simulink model "TEP_Final_NoScript"  (R2024a)
settings: Solver=FixedStepAuto  StartTime=0.0  StopTime=10  FixedStep=1/3600  RelTol=1e-3
model workspace (MAT data in the model file):
  AD : Simulink.Parameter (value not decoded)
  AG : Simulink.Parameter (value not decoded)
  AH : Simulink.Parameter (value not decoded)
  AV : Simulink.Parameter (value not decoded)
  AVP : Simulink.Parameter (value not decoded)
  BCHL : Simulink.Parameter (value not decoded)
  BCHV : Simulink.Parameter (value not decoded)
  BD : Simulink.Parameter (value not decoded)
  BG : Simulink.Parameter (value not decoded)
  BH : Simulink.Parameter (value not decoded)
  BVP : Simulink.Parameter (value not decoded)
  CD : Simulink.Parameter (value not decoded)
  CG : Simulink.Parameter (value not decoded)
  CH : Simulink.Parameter (value not decoded)
  CVP : Simulink.Parameter (value not decoded)
  XMW : Simulink.Parameter (value not decoded)
  XNS : Simulink.Parameter (value not decoded)
  XNSE : Simulink.Parameter (value not decoded)
symbols that are objects in the model workspace (value not decoded): AD, AG, AH, AV, AVP, BD, BG, BH, BVP, CD, CG, CH, CVP, XMW, XNS, XNSE
undefined symbols (not defined in the file or in its folder): magnitude, msgbox, SETPT, XMEAS, XMV
libraries: mylib x360, dspindex x28
(part 8 of 14)

== system TEP_Final_NoScript/Subsystem1/CCin/Subsystem3 ==
  TC : Inport
  P : Inport  Port=2
  Add : Sum  Inputs=+-
  P0 Pa : Constant  Value=1.01325e5
  Subsystem : Subsystem
  Subsystem1 : Subsystem
  Subsystem2 : Subsystem
  T0 K : Constant  Value=298.15
  kPa to Pa : Gain  Gain=1000
  Bph : Outport
  wires:
  kPa to Pa/1 -> Subsystem1/3(P1)
  P0 Pa/1 -> Subsystem1/4(P0)
  Subsystem/1(h-h0 J/mol) -> Add/1
  Subsystem1/1(T0(s-s0) J/mol) -> Add/2
  T0 K/1 -> Subsystem1/2(T0), Subsystem/2(T0)
  Subsystem2/1(TK) -> Subsystem/1(T1), Subsystem1/1(T1)
  TC/1 -> Subsystem2/1(TC)
  Add/1 -> Bph/1
  P/1 -> kPa to Pa/1

== system TEP_Final_NoScript/Subsystem1/CCout/Subsystem ==
  Bph : Inport
  FWR in kg/h : Inport  Port=2
  Gain : Gain  Gain=1/3600
  Product : Product
  kg/kmol : Constant  Value=18.02
  kmol to mol : Gain  Gain=1000
  kmol/h : Product  Inputs=*/
  Bphm J/s : Outport  VectorParamsAs1DForOutWhenUnconnected=off
  wires:
  Product/1 -> Gain/1
  kmol/h/1 -> kmol to mol/1
  Bph/1 -> Product/1
  Gain/1 -> Bphm J/s/1
  kg/kmol/1 -> kmol/h/2
  FWR in kg/h/1 -> kmol/h/1
  kmol to mol/1 -> Product/2

== system TEP_Final_NoScript/Subsystem1/CCout/Subsystem1 ==
  T : Inport
  F : Inport  Port=2
  A : Constant  Value=9.069
  Gain : Gain  Gain=1/3600
  J/mol : Product
  Product : Product
  Product1 : Product
  gpm to lb/h : Constant  Value=500.72
  lb/h to lb-mol/h : Product  Inputs=*/
  lb/lb-mol : Constant  Value=18.02
  mol : Constant  Value=453.59
  mol/h : Product
  Q J/s : Outport  VectorParamsAs1DForOutWhenUnconnected=off
  wires:
  A/1 -> J/mol/1
  mol/1 -> mol/h/1
  lb/lb-mol/1 -> lb/h to lb-mol/h/2
  Product1/1 -> lb/h to lb-mol/h/1
  lb/h to lb-mol/h/1 -> mol/h/2
  Product/1 -> Gain/1
  gpm to lb/h/1 -> Product1/2
  Gain/1 -> Q J/s/1
  mol/h/1 -> Product/2
  J/mol/1 -> Product/1
  T/1 -> J/mol/2
  F/1 -> Product1/1

== system TEP_Final_NoScript/Subsystem1/CCout/Subsystem3 ==
  TC : Inport
  P : Inport  Port=2
  Add : Sum  Inputs=+-
  P0 Pa : Constant  Value=1.01325e5
  Subsystem : Subsystem
  Subsystem1 : Subsystem
  Subsystem2 : Subsystem
  T0 K : Constant  Value=298.15
  kPa to Pa : Gain  Gain=1000
  Bph : Outport
  wires:
  kPa to Pa/1 -> Subsystem1/3(P1)
  P0 Pa/1 -> Subsystem1/4(P0)
  Subsystem/1(h-h0 J/mol) -> Add/1
  Subsystem1/1(T0(s-s0) J/mol) -> Add/2
  T0 K/1 -> Subsystem1/2(T0), Subsystem/2(T0)
  Subsystem2/1(TK) -> Subsystem/1(T1), Subsystem1/1(T1)
  TC/1 -> Subsystem2/1(TC)
  Add/1 -> Bph/1
  P/1 -> kPa to Pa/1

== system TEP_Final_NoScript/Subsystem1/D feed stream/Composition measurement mol% ==
  XST : Inport
  XMNSE : Inport  Port=2
  Bus Creator : BusCreator  Inputs=8
  Subsystem : Subsystem
  SMEASX : Outport
  wires:
  Subsystem/4(SMEASXD) -> Bus Creator/4  "SMEASXD"
  Subsystem/5(SMEASXE) -> Bus Creator/5  "SMEASXE"
  Subsystem/6(SMEASXF) -> Bus Creator/6  "SMEASXF"
  Subsystem/7(SMEASXG) -> Bus Creator/7  "SMEASXG"
  Subsystem/8(SMEASXH) -> Bus Creator/8  "SMEASXH"
  Subsystem/3(SMEASXC) -> Bus Creator/3  "SMEASXC"
  XST/1 -> Subsystem/1(XST)
  Subsystem/2(SMEASXB) -> Bus Creator/2  "SMEASXB"
  Subsystem/1(SMEASXA) -> Bus Creator/1  "SMEASXA"
  Bus Creator/1 -> SMEASX/1  "SMEASX"
  XMNSE/1 -> Subsystem/2(XMNSE)

== system TEP_Final_NoScript/Subsystem1/D feed stream/Flow measurement in kg//h ==
  XMEAS in kg/h : Inport
  "SMEASF " : Outport  VectorParamsAs1DForOutWhenUnconnected=off
  wires:
  XMEAS in kg/h/1 -> "SMEASF "/1

== system TEP_Final_NoScript/Subsystem1/D feed stream/Pressure measurement in kPa ==
  "P in mm Hg " : Inport
  XMNSE : Inport  Port=2
  " kPa" : Constant  Value=101.325
  " mm Hg   " : Constant  Value=760
  Add : Sum
  Pressure conversion kPa : Product  Inputs=*/*
  SMEASP : Outport  VectorParamsAs1DForOutWhenUnconnected=off
  wires:
  "P in mm Hg "/1 -> Pressure conversion kPa/1
  " kPa"/1 -> Pressure conversion kPa/3
  " mm Hg   "/1 -> Pressure conversion kPa/2
  Pressure conversion kPa/1 -> Add/1
  Add/1 -> SMEASP/1  "SMEASP"
  XMNSE/1 -> Add/2

== system TEP_Final_NoScript/Subsystem1/D feed stream/Temperature measurement in C ==
  T in celsius : Inport
  XMNSE : Inport  Port=2
  Add : Sum
  SMEAST : Outport
  wires:
  T in celsius/1 -> Add/1
  Add/1 -> SMEAST/1  "SMEAST"
  XMNSE/1 -> Add/2

== system TEP_Final_NoScript/Subsystem1/E feed stream/Composition measurement mol% ==
  XST : Inport
  XMNSE : Inport  Port=2
  Bus Creator : BusCreator  Inputs=8
  Subsystem : Subsystem
  SMEASX : Outport
  wires:
  Subsystem/4(SMEASXD) -> Bus Creator/4  "SMEASXD"
  Subsystem/5(SMEASXE) -> Bus Creator/5  "SMEASXE"
  Subsystem/6(SMEASXF) -> Bus Creator/6  "SMEASXF"
  Subsystem/7(SMEASXG) -> Bus Creator/7  "SMEASXG"
  Subsystem/8(SMEASXH) -> Bus Creator/8  "SMEASXH"
  Subsystem/3(SMEASXC) -> Bus Creator/3  "SMEASXC"
  XST/1 -> Subsystem/1(XST)
  Subsystem/2(SMEASXB) -> Bus Creator/2  "SMEASXB"
  Subsystem/1(SMEASXA) -> Bus Creator/1  "SMEASXA"
  Bus Creator/1 -> SMEASX/1  "SMEASX"
  XMNSE/1 -> Subsystem/2(XMNSE)

== system TEP_Final_NoScript/Subsystem1/E feed stream/Flow measurement in kg//h ==
  XMEAS in kg/h : Inport
  "SMEASF " : Outport  VectorParamsAs1DForOutWhenUnconnected=off
  wires:
  XMEAS in kg/h/1 -> "SMEASF "/1

== system TEP_Final_NoScript/Subsystem1/E feed stream/Pressure measurement in kPa ==
  "P in mm Hg " : Inport
  XMNSE : Inport  Port=2
  " kPa" : Constant  Value=101.325
  " mm Hg   " : Constant  Value=760
  Add : Sum
  Pressure conversion kPa : Product  Inputs=*/*
  SMEASP : Outport  VectorParamsAs1DForOutWhenUnconnected=off
  wires:
  "P in mm Hg "/1 -> Pressure conversion kPa/1
  " kPa"/1 -> Pressure conversion kPa/3
  " mm Hg   "/1 -> Pressure conversion kPa/2
  Pressure conversion kPa/1 -> Add/1
  Add/1 -> SMEASP/1  "SMEASP"
  XMNSE/1 -> Add/2

== system TEP_Final_NoScript/Subsystem1/E feed stream/Temperature measurement in C ==
  T in celsius : Inport
  XMNSE : Inport  Port=2
  Add : Sum
  SMEAST : Outport
  wires:
  T in celsius/1 -> Add/1
  Add/1 -> SMEAST/1  "SMEAST"
  XMNSE/1 -> Add/2

== system TEP_Final_NoScript/Subsystem1/Product stream/Composition measurement mol% ==
  XST : Inport
  XMNSE2 : Inport  Port=2
  XMNSE3 : Inport  Port=3
  Bus Creator : BusCreator  Inputs=8
  Subsystem : Subsystem
  Subsystem1 : Subsystem
  SMEASX : Outport
  wires:
  Subsystem/3(SMEASXC) -> Bus Creator/3  "SMEASXC"
  XST/1 -> Subsystem1/1(XST), Subsystem/1(XST)
  Subsystem/2(SMEASXB) -> Bus Creator/2  "SMEASXB"
  Subsystem/1(SMEASXA) -> Bus Creator/1  "SMEASXA"
  Bus Creator/1 -> SMEASX/1  "SMEASX"
  XMNSE2/1 -> Subsystem/2(XMNSE)
  Subsystem1/1(SMEASXD) -> Bus Creator/4  "SMEASXD"
  Subsystem1/2(SMEASXE) -> Bus Creator/5  "SMEASXE"
  Subsystem1/3(SMEASXF) -> Bus Creator/6  "SMEASXF"
  Subsystem1/4(SMEASXG) -> Bus Creator/7  "SMEASXG"
  Subsystem1/5(SMEASXH) -> Bus Creator/8  "SMEASXH"
  XMNSE3/1 -> Subsystem1/2(XMNSE3)

== system TEP_Final_NoScript/Subsystem1/Product stream/Flow measurement in kg//h ==
  XMEAS in m^3/h : Inport
  XST : Inport  Port=2
  "       " : Constant  Value=35.3145
  Convert from lb/h to kg/h : Constant  Value=0.454
  XMWS Molecular weight of Stream lb/lb-mol : Subsystem
  kg/h : Product  Inputs=3
  lb-mol/h : Product  Inputs=***
  "SMEASF " : Outport  VectorParamsAs1DForOutWhenUnconnected=off
  wires:
  lb-mol/h/1 -> kg/h/2
  [DLS] -> lb-mol/h/2
  "       "/1 -> lb-mol/h/3
  XMEAS in m^3/h/1 -> lb-mol/h/1
  XMWS Molecular weight of Stream lb/lb-mol/1(XMWS) -> kg/h/1
  Convert from lb/h to kg/h/1 -> kg/h/3
  kg/h/1 -> "SMEASF "/1
  XST/1 -> XMWS Molecular weight of Stream lb/lb-mol/1(XST)

== system TEP_Final_NoScript/Subsystem1/Product stream/Pressure measurement in kPa ==
  "P in mm Hg " : Inport
  XMNSE : Inport  Port=2
  " kPa" : Constant  Value=101.325
  " mm Hg   " : Constant  Value=760
  Add : Sum
  Pressure conversion kPa : Product  Inputs=*/*
  SMEASP : Outport  VectorParamsAs1DForOutWhenUnconnected=off
  wires:
  "P in mm Hg "/1 -> Pressure conversion kPa/1
  " kPa"/1 -> Pressure conversion kPa/3
  " mm Hg   "/1 -> Pressure conversion kPa/2
  Pressure conversion kPa/1 -> Add/1
  Add/1 -> SMEASP/1  "SMEASP"
  XMNSE/1 -> Add/2

== system TEP_Final_NoScript/Subsystem1/Product stream/Temperature measurement in C ==
  XMEAS in celsius : Inport
  SMEAST : Outport
  wires:
  XMEAS in celsius/1 -> SMEAST/1  "SMEAST"

== system TEP_Final_NoScript/Subsystem1/Purge stream/Composition measurement mol% ==
  XMEAS : Inport
  Bus Creator : BusCreator  Inputs=8
  Bus Selector : BusSelector  OutputSignals=XMEAS(29),XMEAS(30),XMEAS(31),XMEAS(32),XMEAS(33),XMEAS(34),XMEAS(35),XMEAS(36)
  SMEASX : Outport
  wires:
  Bus Selector/4 -> Bus Creator/4  "<XMEAS(32)>"
  Bus Selector/5 -> Bus Creator/5  "<XMEAS(33)>"
  Bus Selector/6 -> Bus Creator/6  "<XMEAS(34)>"
  Bus Selector/7 -> Bus Creator/7  "<XMEAS(35)>"
  Bus Selector/8 -> Bus Creator/8  "<XMEAS(36)>"
  Bus Selector/3 -> Bus Creator/3  "<XMEAS(31)>"
  XMEAS/1 -> Bus Selector/1
  Bus Selector/2 -> Bus Creator/2  "<XMEAS(30)>"
  Bus Selector/1 -> Bus Creator/1  "<XMEAS(29)>"
  Bus Creator/1 -> SMEASX/1  "SMEASX"

== system TEP_Final_NoScript/Subsystem1/Purge stream/Flow measurement in kg//h ==
  XMEAS in kscmh : Inport
  XST : Inport  Port=2
  " " : Constant  Value=35.3145
  "  " : Constant  Value=0.359
  Convert from lb/h to kg/h : Constant  Value=0.454
  Product : Product  Inputs=3
  XMWS Molecular weight of Stream lb/lb-mol : Subsystem
  lb-mol/h : Product  Inputs=**/
  "SMEASF " : Outport  VectorParamsAs1DForOutWhenUnconnected=off
  wires:
  " "/1 -> lb-mol/h/2
  "  "/1 -> lb-mol/h/3
  XMEAS in kscmh/1 -> lb-mol/h/1
  Convert from lb/h to kg/h/1 -> Product/3
  XST/1 -> XMWS Molecular weight of Stream lb/lb-mol/1(XST)
  lb-mol/h/1 -> Product/2
  XMWS Molecular weight of Stream lb/lb-mol/1(XMWS) -> Product/1
  Product/1 -> "SMEASF "/1

== system TEP_Final_NoScript/Subsystem1/Purge stream/Pressure measurement in kPa ==
  XMEAS in kPa gauge : Inport
  " kPa" : Constant  Value=101.325
  Add : Sum
  SMEASP : Outport  VectorParamsAs1DForOutWhenUnconnected=off
  wires:
  Add/1 -> SMEASP/1  "SMEASP"
  " kPa"/1 -> Add/2
  XMEAS in kPa gauge/1 -> Add/1

== system TEP_Final_NoScript/Subsystem1/Purge stream/Temperature measurement in C ==
  XMEAS in celsius : Inport
  SMEAST : Outport
  wires:
  XMEAS in celsius/1 -> SMEAST/1  "SMEAST"

== system TEP_Final_NoScript/Subsystem1/RCIn/Flow measurement in kg//h ==
  XMNSE : Inport
  F in gpm : Inport  Port=2
  Add : Sum
  Product : Product
  Product1 : Product
  gpm to lb/h : Constant  Value=500.72
  kg/kmol : Constant  Value=18.02
  kmol : Constant  Value=0.45359237
  kmol/h : Product
  lb/h to lb-mol/h : Product  Inputs=*/
  lb/lb-mol : Constant  Value=18.02
  "SMEASF " : Outport  VectorParamsAs1DForOutWhenUnconnected=off
  wires:
  Add/1 -> "SMEASF "/1  "SMEASF"
  Product/1 -> Add/1
  XMNSE/1 -> Add/2
  Product1/1 -> lb/h to lb-mol/h/1
  lb/lb-mol/1 -> lb/h to lb-mol/h/2
  lb/h to lb-mol/h/1 -> kmol/h/2
  gpm to lb/h/1 -> Product1/2
  F in gpm/1 -> Product1/1
  kmol/1 -> kmol/h/1
  kmol/h/1 -> Product/1
  kg/kmol/1 -> Product/2

== system TEP_Final_NoScript/Subsystem1/RCIn/Pressure measurement in kPa ==
  XMNSE : Inport
  TC : Inport  Port=2
  A Antoine Coefficient A : Constant  Value=11.6834
  Add : Sum
  Add1 : Sum
  Add2 : Sum  Inputs=+-
  B Antoine Coefficient B : Constant  Value=3816.44
  C Antoine Coefficient C : Constant  Value=-46.13
  Divide : Product  Inputs=*/
  Divide1 : Product  Inputs=**
  Math Function : Math  SignedPower=on
  Temperature in Kelvin K : Sum
  To Convert bar to kPa : Constant  Value=100
  To Convert °C to K : Constant  Value=273.15
  SMEASP : Outport  VectorParamsAs1DForOutWhenUnconnected=off
  wires:
  Add/1 -> SMEASP/1  "SMEASP"
  XMNSE/1 -> Add/2
  To Convert °C to K/1 -> Temperature in Kelvin K/2
  TC/1 -> Temperature in Kelvin K/1
  C Antoine Coefficient C/1 -> Add1/1
  Divide/1 -> Add2/2
  B Antoine Coefficient B/1 -> Divide/1
  Add1/1 -> Divide/2
  Math Function/1 -> Divide1/1
  A Antoine Coefficient A/1 -> Add2/1
  Add2/1 -> Math Function/1
  To Convert bar to kPa/1 -> Divide1/2
  Temperature in Kelvin K/1 -> Add1/2
  Divide1/1 -> Add/1

== system TEP_Final_NoScript/Subsystem1/RCIn/Temperature measurement in C ==
  T in celsius : Inport
  XMNSE : Inport  Port=2
  Add : Sum
  SMEAST : Outport
  wires:
  T in celsius/1 -> Add/1
  Add/1 -> SMEAST/1  "SMEAST"
  XMNSE/1 -> Add/2

== system TEP_Final_NoScript/Subsystem1/RCOut/Pressure measurement in kPa ==
  XMNSE : Inport
  TC : Inport  Port=2
  A Antoine Coefficient A : Constant  Value=11.6834
  Add : Sum
  Add1 : Sum
  Add2 : Sum  Inputs=+-
  B Antoine Coefficient B : Constant  Value=3816.44
  C Antoine Coefficient C : Constant  Value=-46.13
  Divide : Product  Inputs=*/
  Divide1 : Product  Inputs=**
  Math Function : Math  SignedPower=on
  Temperature in Kelvin K : Sum
  To Convert bar to kPa : Constant  Value=100
  To Convert °C to K : Constant  Value=273.15
  SMEASP : Outport  VectorParamsAs1DForOutWhenUnconnected=off
  wires:
  Add/1 -> SMEASP/1  "SMEASP"
  XMNSE/1 -> Add/2
  To Convert °C to K/1 -> Temperature in Kelvin K/2
  TC/1 -> Temperature in Kelvin K/1
  C Antoine Coefficient C/1 -> Add1/1
  Divide/1 -> Add2/2
  B Antoine Coefficient B/1 -> Divide/1
  Add1/1 -> Divide/2
  Math Function/1 -> Divide1/1
  A Antoine Coefficient A/1 -> Add2/1
  Add2/1 -> Math Function/1
  To Convert bar to kPa/1 -> Divide1/2
  Temperature in Kelvin K/1 -> Add1/2
  Divide1/1 -> Add/1

== system TEP_Final_NoScript/Subsystem1/RCOut/Temperature measurement in C ==
  T in celsius : Inport
  XMNSE : Inport  Port=2
  Add : Sum
  SMEAST : Outport
  wires:
  T in celsius/1 -> Add/1
  Add/1 -> SMEAST/1  "SMEAST"
  XMNSE/1 -> Add/2

== system TEP_Final_NoScript/Subsystem1/RCin/Subsystem ==
  Bph : Inport
  FWR in kg/h : Inport  Port=2
  Gain : Gain  Gain=1/3600
  Product : Product
  kg/kmol : Constant  Value=18.02
  kmol to mol : Gain  Gain=1000
  kmol/h : Product  Inputs=*/
  Bphm J/s : Outport  VectorParamsAs1DForOutWhenUnconnected=off
  wires:
  Product/1 -> Gain/1
  kmol/h/1 -> kmol to mol/1
  Bph/1 -> Product/1
  Gain/1 -> Bphm J/s/1
  kg/kmol/1 -> kmol/h/2
  FWR in kg/h/1 -> kmol/h/1
  kmol to mol/1 -> Product/2

== system TEP_Final_NoScript/Subsystem1/RCin/Subsystem1 ==
  T : Inport
  F : Inport  Port=2
  A : Constant  Value=9.069
  Gain : Gain  Gain=1/3600
  J/mol : Product
  Product : Product
  Product1 : Product
  gpm to lb/h : Constant  Value=500.72
  lb/h to lb-mol/h : Product  Inputs=*/
  lb/lb-mol : Constant  Value=18.02
  mol : Constant  Value=453.59
  mol/h : Product
  Q J/s : Outport  VectorParamsAs1DForOutWhenUnconnected=off
  wires:
  A/1 -> J/mol/1
  mol/1 -> mol/h/1
  lb/lb-mol/1 -> lb/h to lb-mol/h/2
  Product1/1 -> lb/h to lb-mol/h/1
  lb/h to lb-mol/h/1 -> mol/h/2
  Product/1 -> Gain/1
  gpm to lb/h/1 -> Product1/2
  Gain/1 -> Q J/s/1
  mol/h/1 -> Product/2
  J/mol/1 -> Product/1
  T/1 -> J/mol/2
  F/1 -> Product1/1

== system TEP_Final_NoScript/Subsystem1/RCin/Subsystem3 ==
  TC : Inport
  P : Inport  Port=2
  Add : Sum  Inputs=+-
  P0 Pa : Constant  Value=1.01325e5
  Subsystem : Subsystem
  Subsystem1 : Subsystem
  Subsystem2 : Subsystem
  T0 K : Constant  Value=298.15
  kPa to Pa : Gain  Gain=1000
  Bph : Outport
  wires:
  kPa to Pa/1 -> Subsystem1/3(P1)
  P0 Pa/1 -> Subsystem1/4(P0)
  Subsystem/1(h-h0 J/mol) -> Add/1
  Subsystem1/1(T0(s-s0) J/mol) -> Add/2
  T0 K/1 -> Subsystem1/2(T0), Subsystem/2(T0)
  Subsystem2/1(TK) -> Subsystem/1(T1), Subsystem1/1(T1)
  TC/1 -> Subsystem2/1(TC)
  Add/1 -> Bph/1
  P/1 -> kPa to Pa/1

== system TEP_Final_NoScript/Subsystem1/RCout/Subsystem ==
  Bph : Inport
  FWR in kg/h : Inport  Port=2
  Gain : Gain  Gain=1/3600
  Product : Product
  kg/kmol : Constant  Value=18.02
  kmol to mol : Gain  Gain=1000
  kmol/h : Product  Inputs=*/
  Bphm J/s : Outport  VectorParamsAs1DForOutWhenUnconnected=off
  wires:
  Product/1 -> Gain/1
  kmol/h/1 -> kmol to mol/1
  Bph/1 -> Product/1
  Gain/1 -> Bphm J/s/1
  kg/kmol/1 -> kmol/h/2
  FWR in kg/h/1 -> kmol/h/1
  kmol to mol/1 -> Product/2

== system TEP_Final_NoScript/Subsystem1/RCout/Subsystem1 ==
  T : Inport
  F : Inport  Port=2
  A : Constant  Value=9.069
  Gain : Gain  Gain=1/3600
  J/mol : Product
  Product : Product
  Product1 : Product
  gpm to lb/h : Constant  Value=500.72
  lb/h to lb-mol/h : Product  Inputs=*/
  lb/lb-mol : Constant  Value=18.02
  mol : Constant  Value=453.59
  mol/h : Product
  Q J/s : Outport  VectorParamsAs1DForOutWhenUnconnected=off
  wires:
  A/1 -> J/mol/1
  mol/1 -> mol/h/1
  lb/lb-mol/1 -> lb/h to lb-mol/h/2
  Product1/1 -> lb/h to lb-mol/h/1
  lb/h to lb-mol/h/1 -> mol/h/2
  Product/1 -> Gain/1
  gpm to lb/h/1 -> Product1/2
  Gain/1 -> Q J/s/1
  mol/h/1 -> Product/2
  J/mol/1 -> Product/1
  T/1 -> J/mol/2
  F/1 -> Product1/1

== system TEP_Final_NoScript/Subsystem1/RCout/Subsystem3 ==
  TC : Inport
  P : Inport  Port=2
  Add : Sum  Inputs=+-
  P0 Pa : Constant  Value=1.01325e5
  Subsystem : Subsystem
  Subsystem1 : Subsystem
  Subsystem2 : Subsystem
  T0 K : Constant  Value=298.15
  kPa to Pa : Gain  Gain=1000
  Bph : Outport
  wires:
  kPa to Pa/1 -> Subsystem1/3(P1)
  P0 Pa/1 -> Subsystem1/4(P0)
  Subsystem/1(h-h0 J/mol) -> Add/1
  Subsystem1/1(T0(s-s0) J/mol) -> Add/2
  T0 K/1 -> Subsystem1/2(T0), Subsystem/2(T0)
  Subsystem2/1(TK) -> Subsystem/1(T1), Subsystem1/1(T1)
  TC/1 -> Subsystem2/1(TC)
  Add/1 -> Bph/1
  P/1 -> kPa to Pa/1

== system TEP_Final_NoScript/Subsystem1/Reactor feed stream/Composition measurement mol% ==
  XST : Inport
  XMNSE : Inport  Port=2
  XMEAS : Inport  Port=3
  Bus Creator : BusCreator  Inputs=8
  Subsystem : Subsystem
  SMEASX : Outport
  wires:
  Subsystem/4(SMEASXD) -> Bus Creator/4  "SMEASXD"
  Subsystem/5(SMEASXE) -> Bus Creator/5  "SMEASXE"
  Subsystem/6(SMEASXF) -> Bus Creator/6  "SMEASXF"
  Subsystem/7(SMEASXG) -> Bus Creator/7  "SMEASXG"
  Subsystem/8(SMEASXH) -> Bus Creator/8  "SMEASXH"
  Subsystem/3(SMEASXC) -> Bus Creator/3  "SMEASXC"
  XST/1 -> Subsystem/1(XST)
  Subsystem/2(SMEASXB) -> Bus Creator/2  "SMEASXB"
  Subsystem/1(SMEASXA) -> Bus Creator/1  "SMEASXA"
  Bus Creator/1 -> SMEASX/1  "SMEASX"
  XMNSE/1 -> Subsystem/2(XMNSE)
  XMEAS/1 -> Subsystem/3(XMEAS)

== system TEP_Final_NoScript/Subsystem1/Reactor feed stream/Flow measurement in kg//h ==
  XMEAS in kscmh : Inport
  XST : Inport  Port=2
  " " : Constant  Value=35.3145
  "  " : Constant  Value=0.359
  Convert from lb/h to kg/h : Constant  Value=0.454
  Product : Product  Inputs=3
  XMWS Molecular weight of Stream lb/lb-mol : Subsystem
  lb-mol/h : Product  Inputs=**/
  "SMEASF " : Outport  VectorParamsAs1DForOutWhenUnconnected=off
  wires:
  " "/1 -> lb-mol/h/2
  "  "/1 -> lb-mol/h/3
  XMEAS in kscmh/1 -> lb-mol/h/1
  Convert from lb/h to kg/h/1 -> Product/3
  XST/1 -> XMWS Molecular weight of Stream lb/lb-mol/1(XST)
  lb-mol/h/1 -> Product/2
  XMWS Molecular weight of Stream lb/lb-mol/1(XMWS) -> Product/1
  Product/1 -> "SMEASF "/1

== system TEP_Final_NoScript/Subsystem1/Reactor feed stream/Pressure measurement in kPa ==
  XMEAS in kPa gauge : Inport
  " kPa" : Constant  Value=101.325
  Add : Sum
  SMEASP : Outport  VectorParamsAs1DForOutWhenUnconnected=off
  wires:
  Add/1 -> SMEASP/1  "SMEASP"
  " kPa"/1 -> Add/2
  XMEAS in kPa gauge/1 -> Add/1

== system TEP_Final_NoScript/Subsystem1/Reactor feed stream/Temperature measurement in C ==
  T in celsius : Inport
  XMNSE : Inport  Port=2
  Add : Sum
  SMEAST : Outport
  wires:
  T in celsius/1 -> Add/1
  Add/1 -> SMEAST/1  "SMEAST"
  XMNSE/1 -> Add/2

== system TEP_Final_NoScript/Subsystem1/Reactor product stream/Composition measurement mol% ==
  XST : Inport
  XMNSE : Inport  Port=2
  Bus Creator : BusCreator  Inputs=8
  Subsystem : Subsystem
  SMEASX : Outport
  wires:
  Subsystem/4(SMEASXD) -> Bus Creator/4  "SMEASXD"
  Subsystem/5(SMEASXE) -> Bus Creator/5  "SMEASXE"
  Subsystem/6(SMEASXF) -> Bus Creator/6  "SMEASXF"
  Subsystem/7(SMEASXG) -> Bus Creator/7  "SMEASXG"
  Subsystem/8(SMEASXH) -> Bus Creator/8  "SMEASXH"
  Subsystem/3(SMEASXC) -> Bus Creator/3  "SMEASXC"
  XST/1 -> Subsystem/1(XST)
  Subsystem/2(SMEASXB) -> Bus Creator/2  "SMEASXB"
  Subsystem/1(SMEASXA) -> Bus Creator/1  "SMEASXA"
  Bus Creator/1 -> SMEASX/1  "SMEASX"
  XMNSE/1 -> Subsystem/2(XMNSE)

== system TEP_Final_NoScript/Subsystem1/Reactor product stream/Flow measurement in kg//h ==
  XST : Inport
  XMNSE : Inport  Port=2
  F in lb-mol/h : Inport  Port=3
  Add : Sum
  Convert from lb/h to kg/h : Constant  Value=0.454
  Product : Product  Inputs=3
  XMWS Molecular weight of Stream lb/lb-mol : Subsystem
  "SMEASF " : Outport  VectorParamsAs1DForOutWhenUnconnected=off
  wires:
  Convert from lb/h to kg/h/1 -> Product/3
  Add/1 -> "SMEASF "/1  "SMEASF"
  Product/1 -> Add/1
  XST/1 -> XMWS Molecular weight of Stream lb/lb-mol/1(XST)
  XMWS Molecular weight of Stream lb/lb-mol/1(XMWS) -> Product/1
  XMNSE/1 -> Add/2
  F in lb-mol/h/1 -> Product/2

== system TEP_Final_NoScript/Subsystem1/Reactor product stream/Pressure measurement in kPa ==
  XMEAS in kPa gauge : Inport
  " kPa" : Constant  Value=101.325
  Add : Sum
  SMEASP : Outport  VectorParamsAs1DForOutWhenUnconnected=off
  wires:
  Add/1 -> SMEASP/1  "SMEASP"
  " kPa"/1 -> Add/2
  XMEAS in kPa gauge/1 -> Add/1

== system TEP_Final_NoScript/Subsystem1/Reactor product stream/Temperature measurement in C ==
  XMEAS in celsius : Inport
  SMEAST : Outport
  wires:
  XMEAS in celsius/1 -> SMEAST/1  "SMEAST"

== system TEP_Final_NoScript/Subsystem1/Separator recycle stream/Composition measurement mol% ==
  XST : Inport
  XMNSE : Inport  Port=2
  Bus Creator : BusCreator  Inputs=8
  Subsystem : Subsystem
  SMEASX : Outport
  wires:
  Subsystem/4(SMEASXD) -> Bus Creator/4  "SMEASXD"
  Subsystem/5(SMEASXE) -> Bus Creator/5  "SMEASXE"
  Subsystem/6(SMEASXF) -> Bus Creator/6  "SMEASXF"
  Subsystem/7(SMEASXG) -> Bus Creator/7  "SMEASXG"
  Subsystem/8(SMEASXH) -> Bus Creator/8  "SMEASXH"
  Subsystem/3(SMEASXC) -> Bus Creator/3  "SMEASXC"
  XST/1 -> Subsystem/1(XST)
  Subsystem/2(SMEASXB) -> Bus Creator/2  "SMEASXB"
  Subsystem/1(SMEASXA) -> Bus Creator/1  "SMEASXA"
  Bus Creator/1 -> SMEASX/1  "SMEASX"
  XMNSE/1 -> Subsystem/2(XMNSE)

== system TEP_Final_NoScript/Subsystem1/Separator recycle stream/Flow measurement in kg//h ==
  XMEAS in kscmh : Inport
  XST : Inport  Port=2
  " " : Constant  Value=35.3145
  "  " : Constant  Value=0.359
  Convert from lb/h to kg/h : Constant  Value=0.454
  Product : Product  Inputs=3
  XMWS Molecular weight of Stream lb/lb-mol : Subsystem
  lb-mol/h : Product  Inputs=**/
  "SMEASF " : Outport  VectorParamsAs1DForOutWhenUnconnected=off
  wires:
  " "/1 -> lb-mol/h/2
  "  "/1 -> lb-mol/h/3
  XMEAS in kscmh/1 -> lb-mol/h/1
  Convert from lb/h to kg/h/1 -> Product/3
  XST/1 -> XMWS Molecular weight of Stream lb/lb-mol/1(XST)
  lb-mol/h/1 -> Product/2
  XMWS Molecular weight of Stream lb/lb-mol/1(XMWS) -> Product/1
  Product/1 -> "SMEASF "/1

== system TEP_Final_NoScript/Subsystem1/Separator recycle stream/Pressure measurement in kPa ==
  XMEAS in kPa gauge : Inport
  " kPa" : Constant  Value=101.325
  Add : Sum
  SMEASP : Outport  VectorParamsAs1DForOutWhenUnconnected=off
  wires:
  Add/1 -> SMEASP/1  "SMEASP"
  " kPa"/1 -> Add/2
  XMEAS in kPa gauge/1 -> Add/1

== system TEP_Final_NoScript/Subsystem1/Separator recycle stream/Temperature measurement in C ==
  XMEAS in celsius : Inport
  SMEAST : Outport
  wires:
  XMEAS in celsius/1 -> SMEAST/1  "SMEAST"

== system TEP_Final_NoScript/Subsystem1/Separator underflow stream/Composition measurement mol% ==
  XST : Inport
  XMNSE : Inport  Port=2
  Bus Creator : BusCreator  Inputs=8
  Subsystem : Subsystem
  SMEASX : Outport
  wires:
  Subsystem/4(SMEASXD) -> Bus Creator/4  "SMEASXD"
  Subsystem/5(SMEASXE) -> Bus Creator/5  "SMEASXE"
  Subsystem/6(SMEASXF) -> Bus Creator/6  "SMEASXF"
  Subsystem/7(SMEASXG) -> Bus Creator/7  "SMEASXG"
  Subsystem/8(SMEASXH) -> Bus Creator/8  "SMEASXH"
  Subsystem/3(SMEASXC) -> Bus Creator/3  "SMEASXC"
  XST/1 -> Subsystem/1(XST)
  Subsystem/2(SMEASXB) -> Bus Creator/2  "SMEASXB"
  Subsystem/1(SMEASXA) -> Bus Creator/1  "SMEASXA"
  Bus Creator/1 -> SMEASX/1  "SMEASX"
  XMNSE/1 -> Subsystem/2(XMNSE)

== system TEP_Final_NoScript/Subsystem1/Separator underflow stream/Flow measurement in kg//h ==
  XMEAS in m^3/h : Inport
  XST : Inport  Port=2
  "       " : Constant  Value=35.3145
  Convert from lb/h to kg/h : Constant  Value=0.454
  XMWS Molecular weight of Stream lb/lb-mol : Subsystem
  kg/h : Product  Inputs=3
  lb-mol/h : Product  Inputs=***
  "SMEASF " : Outport  VectorParamsAs1DForOutWhenUnconnected=off
  wires:
  lb-mol/h/1 -> kg/h/2
  [DLS] -> lb-mol/h/2
  "       "/1 -> lb-mol/h/3
  XMEAS in m^3/h/1 -> lb-mol/h/1
  XMWS Molecular weight of Stream lb/lb-mol/1(XMWS) -> kg/h/1
  Convert from lb/h to kg/h/1 -> kg/h/3
  kg/h/1 -> "SMEASF "/1
  XST/1 -> XMWS Molecular weight of Stream lb/lb-mol/1(XST)

== system TEP_Final_NoScript/Subsystem1/Separator underflow stream/Pressure measurement in kPa ==
  "P in mm Hg " : Inport
  XMNSE : Inport  Port=2
  " kPa" : Constant  Value=101.325
  " mm Hg   " : Constant  Value=760
  Add : Sum
  Pressure conversion kPa : Product  Inputs=*/*
  SMEASP : Outport  VectorParamsAs1DForOutWhenUnconnected=off
  wires:
  "P in mm Hg "/1 -> Pressure conversion kPa/1
  " kPa"/1 -> Pressure conversion kPa/3
  " mm Hg   "/1 -> Pressure conversion kPa/2
  Pressure conversion kPa/1 -> Add/1
  Add/1 -> SMEASP/1  "SMEASP"
  XMNSE/1 -> Add/2

== system TEP_Final_NoScript/Subsystem1/Separator underflow stream/Temperature measurement in C ==
  XMEAS in celsius : Inport
  SMEAST : Outport
  wires:
  XMEAS in celsius/1 -> SMEAST/1  "SMEAST"

== system TEP_Final_NoScript/Subsystem1/Stripper recycle stream/Composition measurement mol% ==
  XST : Inport
  XMNSE : Inport  Port=2
  Bus Creator : BusCreator  Inputs=8
  Subsystem : Subsystem
  SMEASX : Outport
  wires:
  Subsystem/4(SMEASXD) -> Bus Creator/4  "SMEASXD"
  Subsystem/5(SMEASXE) -> Bus Creator/5  "SMEASXE"
  Subsystem/6(SMEASXF) -> Bus Creator/6  "SMEASXF"
  Subsystem/7(SMEASXG) -> Bus Creator/7  "SMEASXG"
  Subsystem/8(SMEASXH) -> Bus Creator/8  "SMEASXH"
  Subsystem/3(SMEASXC) -> Bus Creator/3  "SMEASXC"
  XST/1 -> Subsystem/1(XST)
  Subsystem/2(SMEASXB) -> Bus Creator/2  "SMEASXB"
  Subsystem/1(SMEASXA) -> Bus Creator/1  "SMEASXA"
  Bus Creator/1 -> SMEASX/1  "SMEASX"
  XMNSE/1 -> Subsystem/2(XMNSE)

== system TEP_Final_NoScript/Subsystem1/Stripper recycle stream/Flow measurement in kg//h ==
  XST : Inport
  XMNSE : Inport  Port=2
  F in lb-mol/h : Inport  Port=3
  Add : Sum
  Convert from lb/h to kg/h : Constant  Value=0.454
  Product : Product  Inputs=3
  XMWS Molecular weight of Stream lb/lb-mol : Subsystem
  "SMEASF " : Outport  VectorParamsAs1DForOutWhenUnconnected=off
  wires:
  Convert from lb/h to kg/h/1 -> Product/3
  Add/1 -> "SMEASF "/1  "SMEASF"
  Product/1 -> Add/1
  XST/1 -> XMWS Molecular weight of Stream lb/lb-mol/1(XST)
  XMWS Molecular weight of Stream lb/lb-mol/1(XMWS) -> Product/1
  XMNSE/1 -> Add/2
  F in lb-mol/h/1 -> Product/2

== system TEP_Final_NoScript/Subsystem1/Stripper recycle stream/Pressure measurement in kPa ==
  XMEAS in kPa gauge : Inport
  " kPa" : Constant  Value=101.325
  Add : Sum
  SMEASP : Outport  VectorParamsAs1DForOutWhenUnconnected=off
  wires:
  Add/1 -> SMEASP/1  "SMEASP"
  " kPa"/1 -> Add/2
  XMEAS in kPa gauge/1 -> Add/1

== system TEP_Final_NoScript/Subsystem1/Stripper recycle stream/Temperature measurement in C ==
  T in celsius : Inport
  XMNSE : Inport  Port=2
  Add : Sum
  SMEAST : Outport
  wires:
  T in celsius/1 -> Add/1
  Add/1 -> SMEAST/1  "SMEAST"
  XMNSE/1 -> Add/2

== system TEP_Final_NoScript/Subsystem1/Subsystem1/Subsystem1 ==
  SMEASX : Inport
  Bus Creator : BusCreator  Inputs=4
  Bus Selector : BusSelector  OutputSignals=SMEAST,SMEASP,SMEASF,SMEASX
  Composition measurement fraction : Subsystem
  Flow measurement in lb-mol/hr : Subsystem
  Pressure measurement in mmHg : Subsystem
  SMEASXOut : Outport
  wires:
  SMEASX/1 -> Bus Selector/1
  Bus Selector/2 -> Pressure measurement in mmHg/1("P in kPa ")  "<SMEASP>"
  Bus Selector/3 -> Flow measurement in lb-mol/hr/1(F in kg/h)  "<SMEASF>"
  Bus Selector/4 -> Composition measurement fraction/1(X in %)  "<SMEASX>"
  Composition measurement fraction/1(SMEASX) -> Bus Creator/4, Flow measurement in lb-mol/hr/2(XST)  "SMEASX"
  Flow measurement in lb-mol/hr/1("SMEASF ") -> Bus Creator/3  "SMEASF"
  Pressure measurement in mmHg/1(SMEASP) -> Bus Creator/2  "SMEASP"
  Bus Selector/1 -> Bus Creator/1  "<SMEAST>"
  Bus Creator/1 -> SMEASXOut/1

== system TEP_Final_NoScript/Subsystem1/Subsystem13/Subsystem1 ==
  SMEASX : Inport
  Bus Creator : BusCreator  Inputs=4
  Bus Selector : BusSelector  OutputSignals=SMEAST,SMEASP,SMEASF,SMEASX
  Composition measurement fraction : Subsystem
  Flow measurement in lb-mol/hr : Subsystem
  Pressure measurement in mmHg : Subsystem
  SMEASXOut : Outport
  wires:
  SMEASX/1 -> Bus Selector/1
  Bus Selector/2 -> Pressure measurement in mmHg/1("P in kPa ")  "<SMEASP>"
  Bus Selector/3 -> Flow measurement in lb-mol/hr/1(F in kg/h)  "<SMEASF>"
  Bus Selector/4 -> Composition measurement fraction/1(X in %)  "<SMEASX>"
  Composition measurement fraction/1(SMEASX) -> Bus Creator/4, Flow measurement in lb-mol/hr/2(XST)  "SMEASX"
  Flow measurement in lb-mol/hr/1("SMEASF ") -> Bus Creator/3  "SMEASF"
  Pressure measurement in mmHg/1(SMEASP) -> Bus Creator/2  "SMEASP"
  Bus Selector/1 -> Bus Creator/1  "<SMEAST>"
  Bus Creator/1 -> SMEASXOut/1

== system TEP_Final_NoScript/Subsystem1/Subsystem14/Subsystem1 ==
  SMEASX : Inport
  Bus Creator : BusCreator  Inputs=4
  Bus Selector : BusSelector  OutputSignals=SMEAST,SMEASP,SMEASF,SMEASX
  Composition measurement fraction : Subsystem
  Flow measurement in lb-mol/hr : Subsystem
  Pressure measurement in mmHg : Subsystem
  SMEASXOut : Outport
  wires:
  SMEASX/1 -> Bus Selector/1
  Bus Selector/2 -> Pressure measurement in mmHg/1("P in kPa ")  "<SMEASP>"
  Bus Selector/3 -> Flow measurement in lb-mol/hr/1(F in kg/h)  "<SMEASF>"
  Bus Selector/4 -> Composition measurement fraction/1(X in %)  "<SMEASX>"
  Composition measurement fraction/1(SMEASX) -> Bus Creator/4, Flow measurement in lb-mol/hr/2(XST)  "SMEASX"
  Flow measurement in lb-mol/hr/1("SMEASF ") -> Bus Creator/3  "SMEASF"
  Pressure measurement in mmHg/1(SMEASP) -> Bus Creator/2  "SMEASP"
  Bus Selector/1 -> Bus Creator/1  "<SMEAST>"
  Bus Creator/1 -> SMEASXOut/1

== system TEP_Final_NoScript/Subsystem1/Subsystem15/Subsystem1 ==
  SMEASX : Inport
  Bus Creator : BusCreator  Inputs=4
  Bus Selector : BusSelector  OutputSignals=SMEAST,SMEASP,SMEASF,SMEASX
  Composition measurement fraction : Subsystem
  Flow measurement in lb-mol/hr : Subsystem
  Pressure measurement in mmHg : Subsystem
  SMEASXOut : Outport
  wires:
  SMEASX/1 -> Bus Selector/1
  Bus Selector/2 -> Pressure measurement in mmHg/1("P in kPa ")  "<SMEASP>"
  Bus Selector/3 -> Flow measurement in lb-mol/hr/1(F in kg/h)  "<SMEASF>"
  Bus Selector/4 -> Composition measurement fraction/1(X in %)  "<SMEASX>"
  Composition measurement fraction/1(SMEASX) -> Bus Creator/4, Flow measurement in lb-mol/hr/2(XST)  "SMEASX"
  Flow measurement in lb-mol/hr/1("SMEASF ") -> Bus Creator/3  "SMEASF"
  Pressure measurement in mmHg/1(SMEASP) -> Bus Creator/2  "SMEASP"
  Bus Selector/1 -> Bus Creator/1  "<SMEAST>"
  Bus Creator/1 -> SMEASXOut/1

== system TEP_Final_NoScript/Subsystem1/Subsystem16/Subsystem1 ==
  SMEASX : Inport
  Bus Creator : BusCreator  Inputs=4
  Bus Selector : BusSelector  OutputSignals=SMEAST,SMEASP,SMEASF,SMEASX
  Composition measurement fraction : Subsystem
  Flow measurement in lb-mol/hr : Subsystem
  Pressure measurement in mmHg : Subsystem
  SMEASXOut : Outport
  wires:
  SMEASX/1 -> Bus Selector/1
  Bus Selector/2 -> Pressure measurement in mmHg/1("P in kPa ")  "<SMEASP>"
  Bus Selector/3 -> Flow measurement in lb-mol/hr/1(F in kg/h)  "<SMEASF>"
  Bus Selector/4 -> Composition measurement fraction/1(X in %)  "<SMEASX>"
  Composition measurement fraction/1(SMEASX) -> Bus Creator/4, Flow measurement in lb-mol/hr/2(XST)  "SMEASX"
  Flow measurement in lb-mol/hr/1("SMEASF ") -> Bus Creator/3  "SMEASF"
  Pressure measurement in mmHg/1(SMEASP) -> Bus Creator/2  "SMEASP"
  Bus Selector/1 -> Bus Creator/1  "<SMEAST>"
  Bus Creator/1 -> SMEASXOut/1

== system TEP_Final_NoScript/Subsystem1/Subsystem17/Subsystem1 ==
  SMEASX : Inport
  Bus Creator : BusCreator  Inputs=4
  Bus Selector : BusSelector  OutputSignals=SMEAST,SMEASP,SMEASF,SMEASX
  Composition measurement fraction : Subsystem
  Flow measurement in lb-mol/hr : Subsystem
  Pressure measurement in mmHg : Subsystem
  SMEASXOut : Outport
  wires:
  SMEASX/1 -> Bus Selector/1
  Bus Selector/2 -> Pressure measurement in mmHg/1("P in kPa ")  "<SMEASP>"
  Bus Selector/3 -> Flow measurement in lb-mol/hr/1(F in kg/h)  "<SMEASF>"
  Bus Selector/4 -> Composition measurement fraction/1(X in %)  "<SMEASX>"
  Composition measurement fraction/1(SMEASX) -> Bus Creator/4, Flow measurement in lb-mol/hr/2(XST)  "SMEASX"
  Flow measurement in lb-mol/hr/1("SMEASF ") -> Bus Creator/3  "SMEASF"
  Pressure measurement in mmHg/1(SMEASP) -> Bus Creator/2  "SMEASP"
  Bus Selector/1 -> Bus Creator/1  "<SMEAST>"
  Bus Creator/1 -> SMEASXOut/1

== system TEP_Final_NoScript/Subsystem1/Subsystem2/Subsystem1 ==
  SMEASX : Inport
  Bus Creator : BusCreator  Inputs=4
  Bus Selector : BusSelector  OutputSignals=SMEAST,SMEASP,SMEASF,SMEASX
  Composition measurement fraction : Subsystem
  Flow measurement in lb-mol/hr : Subsystem
  Pressure measurement in mmHg : Subsystem
  SMEASXOut : Outport
  wires:
  SMEASX/1 -> Bus Selector/1
  Bus Selector/2 -> Pressure measurement in mmHg/1("P in kPa ")  "<SMEASP>"
  Bus Selector/3 -> Flow measurement in lb-mol/hr/1(F in kg/h)  "<SMEASF>"
  Bus Selector/4 -> Composition measurement fraction/1(X in %)  "<SMEASX>"
  Composition measurement fraction/1(SMEASX) -> Bus Creator/4, Flow measurement in lb-mol/hr/2(XST)  "SMEASX"
  Flow measurement in lb-mol/hr/1("SMEASF ") -> Bus Creator/3  "SMEASF"
  Pressure measurement in mmHg/1(SMEASP) -> Bus Creator/2  "SMEASP"
  Bus Selector/1 -> Bus Creator/1  "<SMEAST>"
  Bus Creator/1 -> SMEASXOut/1

== system TEP_Final_NoScript/Subsystem1/Subsystem3/Subsystem1 ==
  SMEASX : Inport
  Bus Creator : BusCreator  Inputs=4
  Bus Selector : BusSelector  OutputSignals=SMEAST,SMEASP,SMEASF,SMEASX
  Composition measurement fraction : Subsystem
  Flow measurement in lb-mol/hr : Subsystem
  Pressure measurement in mmHg : Subsystem
  SMEASXOut : Outport
  wires:
  SMEASX/1 -> Bus Selector/1
  Bus Selector/2 -> Pressure measurement in mmHg/1("P in kPa ")  "<SMEASP>"
  Bus Selector/3 -> Flow measurement in lb-mol/hr/1(F in kg/h)  "<SMEASF>"
  Bus Selector/4 -> Composition measurement fraction/1(X in %)  "<SMEASX>"
  Composition measurement fraction/1(SMEASX) -> Bus Creator/4, Flow measurement in lb-mol/hr/2(XST)  "SMEASX"
  Flow measurement in lb-mol/hr/1("SMEASF ") -> Bus Creator/3  "SMEASF"
  Pressure measurement in mmHg/1(SMEASP) -> Bus Creator/2  "SMEASP"
  Bus Selector/1 -> Bus Creator/1  "<SMEAST>"
  Bus Creator/1 -> SMEASXOut/1

== system TEP_Final_NoScript/Subsystem1/Subsystem4/Subsystem1 ==
  SMEASX : Inport
  Bus Creator : BusCreator  Inputs=4
  Bus Selector : BusSelector  OutputSignals=SMEAST,SMEASP,SMEASF,SMEASX
  Composition measurement fraction : Subsystem
  Flow measurement in lb-mol/hr : Subsystem
  Pressure measurement in mmHg : Subsystem
  SMEASXOut : Outport
  wires:
  SMEASX/1 -> Bus Selector/1
  Bus Selector/2 -> Pressure measurement in mmHg/1("P in kPa ")  "<SMEASP>"
  Bus Selector/3 -> Flow measurement in lb-mol/hr/1(F in kg/h)  "<SMEASF>"
  Bus Selector/4 -> Composition measurement fraction/1(X in %)  "<SMEASX>"
  Composition measurement fraction/1(SMEASX) -> Bus Creator/4, Flow measurement in lb-mol/hr/2(XST)  "SMEASX"
  Flow measurement in lb-mol/hr/1("SMEASF ") -> Bus Creator/3  "SMEASF"
  Pressure measurement in mmHg/1(SMEASP) -> Bus Creator/2  "SMEASP"
  Bus Selector/1 -> Bus Creator/1  "<SMEAST>"
  Bus Creator/1 -> SMEASXOut/1

== system TEP_Final_NoScript/Subsystem1/Subsystem5/Subsystem1 ==
  SMEASX : Inport
  Bus Creator : BusCreator  Inputs=4
  Bus Selector : BusSelector  OutputSignals=SMEAST,SMEASP,SMEASF,SMEASX
  Composition measurement fraction : Subsystem
  Flow measurement in lb-mol/hr : Subsystem
  Pressure measurement in mmHg : Subsystem
  SMEASXOut : Outport
  wires:
  SMEASX/1 -> Bus Selector/1
  Bus Selector/2 -> Pressure measurement in mmHg/1("P in kPa ")  "<SMEASP>"
  Bus Selector/3 -> Flow measurement in lb-mol/hr/1(F in kg/h)  "<SMEASF>"
  Bus Selector/4 -> Composition measurement fraction/1(X in %)  "<SMEASX>"
  Composition measurement fraction/1(SMEASX) -> Bus Creator/4, Flow measurement in lb-mol/hr/2(XST)  "SMEASX"
  Flow measurement in lb-mol/hr/1("SMEASF ") -> Bus Creator/3  "SMEASF"
  Pressure measurement in mmHg/1(SMEASP) -> Bus Creator/2  "SMEASP"
  Bus Selector/1 -> Bus Creator/1  "<SMEAST>"
  Bus Creator/1 -> SMEASXOut/1

== system TEP_Final_NoScript/Subsystem1/Subsystem8/Subsystem1 ==
  SMEASX : Inport
  Bus Creator : BusCreator  Inputs=4
  Bus Selector : BusSelector  OutputSignals=SMEAST,SMEASP,SMEASF,SMEASX
  Composition measurement fraction : Subsystem
  Flow measurement in lb-mol/hr : Subsystem
  Pressure measurement in mmHg : Subsystem
  SMEASXOut : Outport
  wires:
  SMEASX/1 -> Bus Selector/1
  Bus Selector/2 -> Pressure measurement in mmHg/1("P in kPa ")  "<SMEASP>"
  Bus Selector/3 -> Flow measurement in lb-mol/hr/1(F in kg/h)  "<SMEASF>"
  Bus Selector/4 -> Composition measurement fraction/1(X in %)  "<SMEASX>"
  Composition measurement fraction/1(SMEASX) -> Bus Creator/4, Flow measurement in lb-mol/hr/2(XST)  "SMEASX"
  Flow measurement in lb-mol/hr/1("SMEASF ") -> Bus Creator/3  "SMEASF"
  Pressure measurement in mmHg/1(SMEASP) -> Bus Creator/2  "SMEASP"
  Bus Selector/1 -> Bus Creator/1  "<SMEAST>"
  Bus Creator/1 -> SMEASXOut/1

== system TEP_Final_NoScript/Mixing Zone/Stream 6/Subsystem/If Action Subsystem ==
  In1 : Inport
  Action Port : ActionPort  ActionPortLabel=if(u1 < 0)
  Out1 : Outport  VectorParamsAs1DForOutWhenUnconnected=off
  wires:
  In1/1 -> Out1/1

== system TEP_Final_NoScript/Mixing Zone/Stream 6/Subsystem/If Action Subsystem1 ==
  In1 : Inport
  Action Port : ActionPort  ActionPortLabel=else
  Out1 : Outport  VectorParamsAs1DForOutWhenUnconnected=off
  wires:
  In1/1 -> Out1/1

== system TEP_Final_NoScript/Process Measurements/Feed Streams/D Feed/XMWS(1) Molecular weight of Stream 1 lb//lb-mol ==
  XST(I,1) : Inport
  Product : Product
  Sum of Elements : Sum  Inputs=+
  "XMW(I) Molecular weight of components lb/lb-mol " : Constant  Value=XMW
  XMWS(1) : Outport  VectorParamsAs1DForOutWhenUnconnected=off
  wires:
  Sum of Elements/1 -> XMWS(1)/1
  Product/1 -> Sum of Elements/1
  XST(I,1)/1 -> Product/1
  "XMW(I) Molecular weight of components lb/lb-mol "/1 -> Product/2

== system TEP_Final_NoScript/Process Measurements/Feed Streams/E Feed/XMWS(2) Molecular weight of Stream 2 lb//lb-mol ==
  XST(I,2) : Inport
  Product : Product
  Sum of Elements : Sum  Inputs=+
  "XMW(I) Molecular weight of components lb/lb-mol " : Constant  Value=XMW
  XMWS(2) : Outport  VectorParamsAs1DForOutWhenUnconnected=off
  wires:
  Sum of Elements/1 -> XMWS(2)/1
  Product/1 -> Sum of Elements/1
  XST(I,2)/1 -> Product/1
  "XMW(I) Molecular weight of components lb/lb-mol "/1 -> Product/2

== system TEP_Final_NoScript/Process Measurements/Product analysis/Subsystem/Subsystem ==
  XST : Inport
  Constant : Constant  Value=100
  Multiport Selector : dspindex/Multiport Selector  rowsOrCols=Rows  idxCellArray={4,5,6,7,8}  idxErrMode=Clip Index
  XCMP(37) : Product
  XCMP(38) : Product
  XCMP(39) : Product
  XCMP(40) : Product
  XCMP(41) : Product
  "XCMP(37) " : Outport  VectorParamsAs1DForOutWhenUnconnected=off
  "XCMP(38) " : Outport  Port=2  VectorParamsAs1DForOutWhenUnconnected=off
  "XCMP(39) " : Outport  Port=3  VectorParamsAs1DForOutWhenUnconnected=off
  "XCMP(40) " : Outport  Port=4  VectorParamsAs1DForOutWhenUnconnected=off
  "XCMP(41) " : Outport  Port=5  VectorParamsAs1DForOutWhenUnconnected=off
  wires:
  Constant/1 -> XCMP(38)/2, XCMP(40)/2, XCMP(41)/2, XCMP(39)/2, XCMP(37)/2
  Multiport Selector/1 -> XCMP(37)/1
  XCMP(37)/1 -> "XCMP(37) "/1  "XCMP(37)"
  Multiport Selector/5 -> XCMP(41)/1
  XCMP(39)/1 -> "XCMP(39) "/1  "XCMP(39)"
  XST/1 -> Multiport Selector/1
  Multiport Selector/4 -> XCMP(40)/1
  Multiport Selector/2 -> XCMP(38)/1
  Multiport Selector/3 -> XCMP(39)/1
  XCMP(38)/1 -> "XCMP(38) "/1  "XCMP(38)"
  XCMP(41)/1 -> "XCMP(41) "/1  "XCMP(41)"
  XCMP(40)/1 -> "XCMP(40) "/1  "XCMP(40)"

== system TEP_Final_NoScript/Process Measurements/Purge gas analysis/Subsystem/Subsystem ==
  XST : Inport
  Constant : Constant  Value=100
  Multiport Selector : dspindex/Multiport Selector  rowsOrCols=Rows  idxCellArray={ 1,2,3,4,5,6,7,8}  idxErrMode=Clip Index
  XCMP(29) : Product
  XCMP(30) : Product
  XCMP(31) : Product
  XCMP(32) : Product
  XCMP(33) : Product
  XCMP(34) : Product
  XCMP(35) : Product
  XCMP(36) : Product
  "XCMP(29) " : Outport  VectorParamsAs1DForOutWhenUnconnected=off
  "XCMP(30) " : Outport  Port=2  VectorParamsAs1DForOutWhenUnconnected=off
  "XCMP(31) " : Outport  Port=3  VectorParamsAs1DForOutWhenUnconnected=off
  "XCMP(32) " : Outport  Port=4  VectorParamsAs1DForOutWhenUnconnected=off
  "XCMP(33) " : Outport  Port=5  VectorParamsAs1DForOutWhenUnconnected=off
  "XCMP(34) " : Outport  Port=6  VectorParamsAs1DForOutWhenUnconnected=off
  "XCMP(35) " : Outport  Port=7  VectorParamsAs1DForOutWhenUnconnected=off
  "XCMP(36) " : Outport  Port=8  VectorParamsAs1DForOutWhenUnconnected=off
  wires:
  XCMP(32)/1 -> "XCMP(32) "/1  "XCMP(32)"
  Multiport Selector/6 -> XCMP(34)/1
  Multiport Selector/8 -> XCMP(36)/1
  XCMP(29)/1 -> "XCMP(29) "/1  "XCMP(29)"
  Multiport Selector/5 -> XCMP(33)/1
  Multiport Selector/7 -> XCMP(35)/1
  XCMP(30)/1 -> "XCMP(30) "/1  "XCMP(30)"
  Multiport Selector/1 -> XCMP(29)/1
  Multiport Selector/3 -> XCMP(31)/1
  Constant/1 -> XCMP(32)/2, XCMP(36)/2, XCMP(35)/2, XCMP(34)/2, XCMP(33)/2, XCMP(31)/2, XCMP(30)/2, XCMP(29)/2
  XCMP(33)/1 -> "XCMP(33) "/1  "XCMP(33)"
  Multiport Selector/4 -> XCMP(32)/1
  XST/1 -> Multiport Selector/1
  Multiport Selector/2 -> XCMP(30)/1
  XCMP(31)/1 -> "XCMP(31) "/1  "XCMP(31)"
  XCMP(35)/1 -> "XCMP(35) "/1  "XCMP(35)"
  XCMP(36)/1 -> "XCMP(36) "/1  "XCMP(36)"
  XCMP(34)/1 -> "XCMP(34) "/1  "XCMP(34)"

== system TEP_Final_NoScript/Process Measurements/Reactor feed analysis/Subsystem/Subsystem ==
  XST : Inport
  Constant : Constant  Value=100
  Multiport Selector : dspindex/Multiport Selector  rowsOrCols=Rows  idxCellArray={ 1,2,3,4,5,6,}  idxErrMode=Clip Index
  XCMP(23) : Product
  XCMP(24) : Product
  XCMP(25) : Product
  XCMP(26) : Product
  XCMP(27) : Product
  XCMP(28) : Product
  XCMP(23)1 : Outport  VectorParamsAs1DForOutWhenUnconnected=off
  XCMP(24)1 : Outport  Port=2  VectorParamsAs1DForOutWhenUnconnected=off
  XCMP(25)1 : Outport  Port=3  VectorParamsAs1DForOutWhenUnconnected=off
  XCMP(26)1 : Outport  Port=4  VectorParamsAs1DForOutWhenUnconnected=off
  XCMP(27)1 : Outport  Port=5  VectorParamsAs1DForOutWhenUnconnected=off
  XCMP(28)1 : Outport  Port=6  VectorParamsAs1DForOutWhenUnconnected=off
  wires:
  Multiport Selector/1 -> XCMP(23)/1  "XST(1;7)"
  Multiport Selector/4 -> XCMP(26)/1  "XST(4;7)"
  Constant/1 -> XCMP(26)/2, XCMP(28)/2, XCMP(27)/2, XCMP(25)/2, XCMP(24)/2, XCMP(23)/2
  Multiport Selector/2 -> XCMP(24)/1  "XST(2;7)"
  XST/1 -> Multiport Selector/1
  Multiport Selector/6 -> XCMP(28)/1  "XST(6:7)"
  Multiport Selector/3 -> XCMP(25)/1  "XST(3;7)"
  XCMP(23)/1 -> XCMP(23)1/1  "XCMP(23)"
  Multiport Selector/5 -> XCMP(27)/1  "XST(5;7)"
  XCMP(25)/1 -> XCMP(25)1/1  "XCMP(25)"
  XCMP(26)/1 -> XCMP(26)1/1  "XCMP(26)"
  XCMP(24)/1 -> XCMP(24)1/1  "XCMP(24)"
  XCMP(27)/1 -> XCMP(27)1/1  "XCMP(27)"
  XCMP(28)/1 -> XCMP(28)1/1  "XCMP(28)"

== system TEP_Final_NoScript/Random number generator1/Disturbances I=1-9/Subsystem1/DIST(2)_0 ==
  BDIST(2) : Constant  Value=0
  Bus Creator : BusCreator  Inputs=6
  CDIST(2) : Constant  Value=0
  DDIST(2) : Constant  Value=0
  SZERO(2) : Constant  Value=0.005
  TENXT(2) : Constant  Value=0.1
  TLAST(2) : Constant  Value=0
  DIST : Outport  VectorParamsAs1DForOutWhenUnconnected=off
  wires:
  Bus Creator/1 -> DIST/1
  TENXT(2)/1 -> Bus Creator/5  "TNEXT"
  SZERO(2)/1 -> Bus Creator/1  "ADIST"
  TLAST(2)/1 -> Bus Creator/6  "TLAST"
  DDIST(2)/1 -> Bus Creator/4  "DDIST"
  BDIST(2)/1 -> Bus Creator/2  "BDIST"
  CDIST(2)/1 -> Bus Creator/3  "CDIST"

== system TEP_Final_NoScript/Random number generator1/Disturbances I=1-9/Subsystem1/Subsystem ==
  Bus Creator : BusCreator  Inputs=5
  HSPAN(2) : Constant  Value=0.7
  HZERO(2) : Constant
  SPSPAN(2) : Constant  Value=0
  SSPAN(2) : Constant  Value=0.003
  SZERO(2) : Constant  Value=0.005
  Out1 : Outport  VectorParamsAs1DForOutWhenUnconnected=off
  wires:
  SSPAN(2)/1 -> Bus Creator/3  "SSPAN"
  HSPAN(2)/1 -> Bus Creator/1  "HSPAN"
  Bus Creator/1 -> Out1/1
  SPSPAN(2)/1 -> Bus Creator/5  "SPSPAN"
  HZERO(2)/1 -> Bus Creator/2  "HZERO"
  SZERO(2)/1 -> Bus Creator/4  "SZERO"

== system TEP_Final_NoScript/Random number generator1/Disturbances I=1-9/Subsystem10/DIST(1)_0 ==
  BDIST(1) : Constant  Value=0
  Bus Creator : BusCreator  Inputs=6
  CDIST(1) : Constant  Value=0
  DDIST(1) : Constant  Value=0
  SZERO(1) : Constant  Value=0.485
  TENXT(1) : Constant  Value=0.1
  TLAST(1) : Constant  Value=0
  DIST : Outport  VectorParamsAs1DForOutWhenUnconnected=off
  wires:
  Bus Creator/1 -> DIST/1
  TENXT(1)/1 -> Bus Creator/5  "TNEXT"
  SZERO(1)/1 -> Bus Creator/1  "ADIST"
  TLAST(1)/1 -> Bus Creator/6  "TLAST"
  DDIST(1)/1 -> Bus Creator/4  "DDIST"
  BDIST(1)/1 -> Bus Creator/2  "BDIST"
  CDIST(1)/1 -> Bus Creator/3  "CDIST"

== system TEP_Final_NoScript/Random number generator1/Disturbances I=1-9/Subsystem10/Subsystem ==
  Bus Creator : BusCreator  Inputs=5
  HSPAN(1) : Constant  Value=0.2
  HZERO(1) : Constant  Value=0.5
  SPSPAN(1) : Constant  Value=0
  SSPAN(1) : Constant  Value=0.03
  SZERO(1) : Constant  Value=0.485
  Out1 : Outport  VectorParamsAs1DForOutWhenUnconnected=off
  wires:
  SSPAN(1)/1 -> Bus Creator/3  "SSPAN"
  HSPAN(1)/1 -> Bus Creator/1  "HSPAN"
  Bus Creator/1 -> Out1/1
  SPSPAN(1)/1 -> Bus Creator/5  "SPSPAN"
  HZERO(1)/1 -> Bus Creator/2  "HZERO"
  SZERO(1)/1 -> Bus Creator/4  "SZERO"

== system TEP_Final_NoScript/Random number generator1/Disturbances I=1-9/Subsystem2/DIST(3)_0 ==
  BDIST(3) : Constant  Value=0
  Bus Creator : BusCreator  Inputs=6
  CDIST(3) : Constant  Value=0
  DDIST(3) : Constant  Value=0
  SZERO(3) : Constant  Value=45
  TENXT(3) : Constant  Value=0.1
  TLAST(3) : Constant  Value=0
  DIST : Outport  VectorParamsAs1DForOutWhenUnconnected=off
  wires:
  Bus Creator/1 -> DIST/1
  TENXT(3)/1 -> Bus Creator/5  "TNEXT"
  SZERO(3)/1 -> Bus Creator/1  "ADIST"
  TLAST(3)/1 -> Bus Creator/6  "TLAST"
  DDIST(3)/1 -> Bus Creator/4  "DDIST"
  BDIST(3)/1 -> Bus Creator/2  "BDIST"
  CDIST(3)/1 -> Bus Creator/3  "CDIST"

== system TEP_Final_NoScript/Random number generator1/Disturbances I=1-9/Subsystem2/Subsystem ==
  Bus Creator : BusCreator  Inputs=5
  HSPAN(3) : Constant  Value=0.25
  HZERO(3) : Constant  Value=0.5
  SPSPAN(3) : Constant  Value=0
  SSPAN(3) : Constant  Value=10
  SZERO(3) : Constant  Value=45
  Out1 : Outport  VectorParamsAs1DForOutWhenUnconnected=off
  wires:
  SSPAN(3)/1 -> Bus Creator/3  "SSPAN"
  HSPAN(3)/1 -> Bus Creator/1  "HSPAN"
  Bus Creator/1 -> Out1/1
  SPSPAN(3)/1 -> Bus Creator/5  "SPSPAN"
  HZERO(3)/1 -> Bus Creator/2  "HZERO"
  SZERO(3)/1 -> Bus Creator/4  "SZERO"

== system TEP_Final_NoScript/Random number generator1/Disturbances I=1-9/Subsystem3/DIST(4)_0 ==
  BDIST(4) : Constant  Value=0
  Bus Creator : BusCreator  Inputs=6
  CDIST(4) : Constant  Value=0
  DDIST(4) : Constant  Value=0
  SZERO(4) : Constant  Value=45
  TENXT(4) : Constant  Value=0.1
  TLAST(4) : Constant  Value=0
  DIST : Outport  VectorParamsAs1DForOutWhenUnconnected=off
  wires:
  Bus Creator/1 -> DIST/1
  TENXT(4)/1 -> Bus Creator/5  "TNEXT"
  SZERO(4)/1 -> Bus Creator/1  "ADIST"
  TLAST(4)/1 -> Bus Creator/6  "TLAST"
  DDIST(4)/1 -> Bus Creator/4  "DDIST"
  BDIST(4)/1 -> Bus Creator/2  "BDIST"
  CDIST(4)/1 -> Bus Creator/3  "CDIST"
